simulink model "computeH"  (Simulink 7.7)
settings: Solver=FixedStepDiscrete  StartTime=0.0  StopTime=100.0  FixedStep=Ts  RelTol=1e-3
InitFcn:
  | robotName = 'icubGazeboSim';
  | localName = 'SimulinkiCubGazeboSim';
  | Ts = 0.1;
libraries: WBCLibrary x7
settings Model: Creator=iron  LastModifiedBy=iron

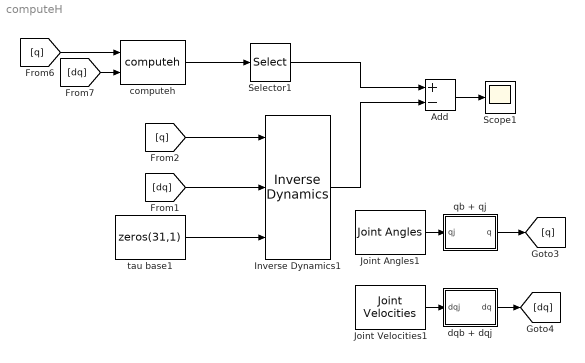
== system computeH ==
  Add : Sum  Inputs=+-
  Inverse Dynamics1 : WBCLibrary/wholeBodyModel/Dynamics/Inverse Dynamics  SystemSampleTime=-1  robotName=robotName  localName=localName
  Joint Angles1 : WBCLibrary/wholeBodyStates/Joint Angles  SystemSampleTime=-1  robotName=robotName  localName=localName
  Joint Velocities1 : WBCLibrary/wholeBodyStates/Joint Velocities  SystemSampleTime=-1  robotName=robotName  localName=localName
  Scope1 : Scope
      settings: TimeRange=10  YMin=-0.1  YMax=0.175
  Selector1 : Selector  InputPortWidth=31  IndexOptions=Index vector (dialog)  Indices=[7:31]  OutputSizes=1
  computeh : WBCLibrary/wholeBodyModel/Dynamics/computeh  SystemSampleTime=-1  val=7  robotname=robotName  localname=localName
  dqb + dqj : Subsystem
  qb + qj : Subsystem
  tau base1 : Constant  Value=zeros(31,1)
  wires:
  [q] -> Inverse Dynamics1/1
  [dq] -> Inverse Dynamics1/2
  tau base1/1 -> Inverse Dynamics1/3
  computeh/1 -> Selector1/1
  Selector1/1 -> Add/1
  Inverse Dynamics1/1 -> Add/2
  Add/1 -> Scope1/1
  [q] -> computeh/1
  [dq] -> computeh/2
  Joint Angles1/1 -> qb + qj/1(qj)
  qb + qj/1(q) -> [q]
  Joint Velocities1/1 -> dqb + dqj/1(dqj)
  dqb + dqj/1(dq) -> [dq]

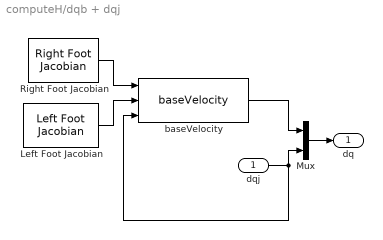
== system computeH/dqb + dqj ==
  dqj : Inport
  Left Foot Jacobian : WBCLibrary/wholeBodyModel/Jacobians/Left Foot Jacobian  SystemSampleTime=-1  robotName=robotName  localName=localName
  Mux : Mux  Inputs=2
  Right Foot Jacobian : WBCLibrary/wholeBodyModel/Jacobians/Right Foot Jacobian  SystemSampleTime=-1  robotName=robotName  localName=localName
  baseVelocity : WBCLibrary/Utilities/baseVelocity  SystemSampleTime=-1
  dq : Outport
  wires:
  Left Foot Jacobian/1 -> baseVelocity/2
  Right Foot Jacobian/1 -> baseVelocity/1
  baseVelocity/1 -> Mux/1
  dqj/1 -> baseVelocity/3, Mux/2
  Mux/1 -> dq/1

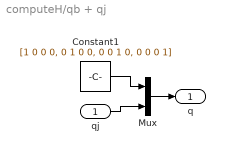
== system computeH/qb + qj ==
  qj : Inport
  Constant1 : Constant  Value=[1 0 0 0, 0 1 0 0, 0 0 1 0, 0 0 0 1]
  Mux : Mux  Inputs=2
  q : Outport
  wires:
  Mux/1 -> q/1
  Constant1/1 -> Mux/1
  qj/1 -> Mux/2
